simulink model "NUgus_servo"  (R2019a)
settings: Solver=VariableStepAuto  StartTime=0.0  StopTime=10  RelTol=1e-3
values from neighbouring files (symbols this model uses):
  head = [-0.05482228998067195, -0.00010888238321339966, 0.0011712900228573724, 0.41900000000000004]    [comtest.m]
  s = mean(abs(present_speed.data))    [RunServoTest.m]
  torso = [0.0050079703254699804, 0.008880921777563762, 0.1021503146237477, 2.5390000000000006]    [comtest.m]
undefined symbols (not defined in the file or in its folder): floor, X, Y, Z
libraries: sm_lib x206, fl_ps_legacy_lib x120, nesl_utility x62, fl_lib x8
(part 8 of 8)

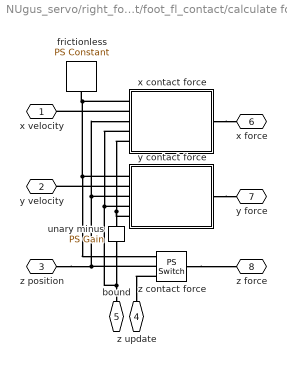
== system NUgus_servo/right_foot/foot_fl_contact/calculate forces ==
  frictionless : fl_lib/Physical Signals/Sources/PS Constant  constant=0
  unary minus : fl_ps_legacy_lib/Legacy Physical Signals/Functions/PS Gain  gain=-1
      settings: SourceProductName=Simscape
  x contact force : Subsystem
  y contact force : Subsystem
  z contact force : fl_ps_legacy_lib/Legacy Physical Signals/Nonlinear Operators/PS Switch  Threshold=0
      settings: SourceProductName=Simscape  SourceProductBaseCode=SS
  x velocity : PMIOPort  Side=Left
  y velocity : PMIOPort  Port=2  Side=Left
  z position : PMIOPort  Port=3  Side=Left
  z update : PMIOPort  Port=4  Side=Left
  bound : PMIOPort  Port=5  Side=Left
  x force : PMIOPort  Port=6  Side=Right
  y force : PMIOPort  Port=7  Side=Right
  z force : PMIOPort  Port=8  Side=Right
  connections:
  x contact force/LConn2 -- x velocity/RConn1
  y contact force/LConn2 -- y velocity/RConn1
  y contact force/RConn1 -- y force/RConn1
  x contact force/RConn1 -- x force/RConn1
  z contact force/RConn1 -- z force/RConn1
  y contact force/LConn3 -- x contact force/LConn3 -- z position/RConn1 -- z contact force/LConn2
  y contact force/LConn4 -- x contact force/LConn4 -- unary minus/LConn1 -- bound/RConn1
  y contact force/LConn5 -- x contact force/LConn5 -- unary minus/RConn1
  x contact force/LConn1 -- frictionless/RConn1 -- y contact force/LConn1 -- z contact force/LConn1
  z contact force/LConn3 -- z update/RConn1

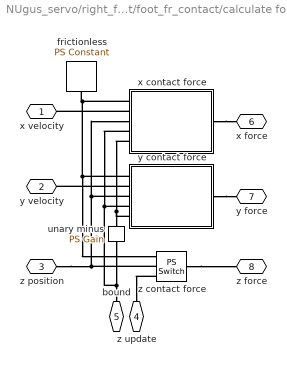
== system NUgus_servo/right_foot/foot_fr_contact/calculate forces ==
  frictionless : fl_lib/Physical Signals/Sources/PS Constant  constant=0
  unary minus : fl_ps_legacy_lib/Legacy Physical Signals/Functions/PS Gain  gain=-1
      settings: SourceProductName=Simscape
  x contact force : Subsystem
  y contact force : Subsystem
  z contact force : fl_ps_legacy_lib/Legacy Physical Signals/Nonlinear Operators/PS Switch  Threshold=0
      settings: SourceProductName=Simscape  SourceProductBaseCode=SS
  x velocity : PMIOPort  Side=Left
  y velocity : PMIOPort  Port=2  Side=Left
  z position : PMIOPort  Port=3  Side=Left
  z update : PMIOPort  Port=4  Side=Left
  bound : PMIOPort  Port=5  Side=Left
  x force : PMIOPort  Port=6  Side=Right
  y force : PMIOPort  Port=7  Side=Right
  z force : PMIOPort  Port=8  Side=Right
  connections:
  x contact force/LConn2 -- x velocity/RConn1
  y contact force/LConn2 -- y velocity/RConn1
  y contact force/RConn1 -- y force/RConn1
  x contact force/RConn1 -- x force/RConn1
  z contact force/RConn1 -- z force/RConn1
  y contact force/LConn3 -- x contact force/LConn3 -- z position/RConn1 -- z contact force/LConn2
  y contact force/LConn4 -- x contact force/LConn4 -- unary minus/LConn1 -- bound/RConn1
  y contact force/LConn5 -- x contact force/LConn5 -- unary minus/RConn1
  x contact force/LConn1 -- frictionless/RConn1 -- y contact force/LConn1 -- z contact force/LConn1
  z contact force/LConn3 -- z update/RConn1

== system NUgus_servo/left_foot/foot_bl_contact/calculate forces/x contact force ==
  PS Max : fl_ps_legacy_lib/Legacy Physical Signals/Nonlinear Operators/PS Max
      settings: SourceProductName=Simscape  SourceProductBaseCode=SS
  PS Min : fl_ps_legacy_lib/Legacy Physical Signals/Nonlinear Operators/PS Min
      settings: SourceProductName=Simscape  SourceProductBaseCode=SS
  PS Switch1 : fl_ps_legacy_lib/Legacy Physical Signals/Nonlinear Operators/PS Switch  Threshold=0
      settings: SourceProductName=Simscape  SourceProductBaseCode=SS
  frictionless : PMIOPort  Side=Left
  force : PMIOPort  Port=2  Side=Right
  velocity : PMIOPort  Port=3  Side=Left
  z position : PMIOPort  Port=4  Side=Left
  upper_bound : PMIOPort  Port=5  Side=Left
  lower_bound : PMIOPort  Port=6  Side=Left
  connections:
  PS Max/LConn2 -- lower_bound/RConn1
  PS Max/LConn1 -- PS Min/RConn1
  PS Switch1/LConn3 -- PS Max/RConn1
  PS Min/LConn1 -- velocity/RConn1
  z position/RConn1 -- PS Switch1/LConn2
  PS Switch1/LConn1 -- frictionless/RConn1
  PS Switch1/RConn1 -- force/RConn1
  PS Min/LConn2 -- upper_bound/RConn1

== system NUgus_servo/left_foot/foot_bl_contact/calculate forces/y contact force ==
  PS Max : fl_ps_legacy_lib/Legacy Physical Signals/Nonlinear Operators/PS Max
      settings: SourceProductName=Simscape  SourceProductBaseCode=SS
  PS Min : fl_ps_legacy_lib/Legacy Physical Signals/Nonlinear Operators/PS Min
      settings: SourceProductName=Simscape  SourceProductBaseCode=SS
  PS Switch1 : fl_ps_legacy_lib/Legacy Physical Signals/Nonlinear Operators/PS Switch  Threshold=0
      settings: SourceProductName=Simscape  SourceProductBaseCode=SS
  frictionless : PMIOPort  Side=Left
  force : PMIOPort  Port=2  Side=Right
  velocity : PMIOPort  Port=3  Side=Left
  z position : PMIOPort  Port=4  Side=Left
  upper_bound : PMIOPort  Port=5  Side=Left
  lower_bound : PMIOPort  Port=6  Side=Left
  connections:
  PS Max/LConn2 -- lower_bound/RConn1
  PS Max/LConn1 -- PS Min/RConn1
  PS Switch1/LConn3 -- PS Max/RConn1
  PS Min/LConn1 -- velocity/RConn1
  z position/RConn1 -- PS Switch1/LConn2
  PS Switch1/LConn1 -- frictionless/RConn1
  PS Switch1/RConn1 -- force/RConn1
  PS Min/LConn2 -- upper_bound/RConn1

== system NUgus_servo/left_foot/foot_br_contact/calculate forces/x contact force ==
  PS Max : fl_ps_legacy_lib/Legacy Physical Signals/Nonlinear Operators/PS Max
      settings: SourceProductName=Simscape  SourceProductBaseCode=SS
  PS Min : fl_ps_legacy_lib/Legacy Physical Signals/Nonlinear Operators/PS Min
      settings: SourceProductName=Simscape  SourceProductBaseCode=SS
  PS Switch1 : fl_ps_legacy_lib/Legacy Physical Signals/Nonlinear Operators/PS Switch  Threshold=0
      settings: SourceProductName=Simscape  SourceProductBaseCode=SS
  frictionless : PMIOPort  Side=Left
  force : PMIOPort  Port=2  Side=Right
  velocity : PMIOPort  Port=3  Side=Left
  z position : PMIOPort  Port=4  Side=Left
  upper_bound : PMIOPort  Port=5  Side=Left
  lower_bound : PMIOPort  Port=6  Side=Left
  connections:
  PS Max/LConn2 -- lower_bound/RConn1
  PS Max/LConn1 -- PS Min/RConn1
  PS Switch1/LConn3 -- PS Max/RConn1
  PS Min/LConn1 -- velocity/RConn1
  z position/RConn1 -- PS Switch1/LConn2
  PS Switch1/LConn1 -- frictionless/RConn1
  PS Switch1/RConn1 -- force/RConn1
  PS Min/LConn2 -- upper_bound/RConn1

== system NUgus_servo/left_foot/foot_br_contact/calculate forces/y contact force ==
  PS Max : fl_ps_legacy_lib/Legacy Physical Signals/Nonlinear Operators/PS Max
      settings: SourceProductName=Simscape  SourceProductBaseCode=SS
  PS Min : fl_ps_legacy_lib/Legacy Physical Signals/Nonlinear Operators/PS Min
      settings: SourceProductName=Simscape  SourceProductBaseCode=SS
  PS Switch1 : fl_ps_legacy_lib/Legacy Physical Signals/Nonlinear Operators/PS Switch  Threshold=0
      settings: SourceProductName=Simscape  SourceProductBaseCode=SS
  frictionless : PMIOPort  Side=Left
  force : PMIOPort  Port=2  Side=Right
  velocity : PMIOPort  Port=3  Side=Left
  z position : PMIOPort  Port=4  Side=Left
  upper_bound : PMIOPort  Port=5  Side=Left
  lower_bound : PMIOPort  Port=6  Side=Left
  connections:
  PS Max/LConn2 -- lower_bound/RConn1
  PS Max/LConn1 -- PS Min/RConn1
  PS Switch1/LConn3 -- PS Max/RConn1
  PS Min/LConn1 -- velocity/RConn1
  z position/RConn1 -- PS Switch1/LConn2
  PS Switch1/LConn1 -- frictionless/RConn1
  PS Switch1/RConn1 -- force/RConn1
  PS Min/LConn2 -- upper_bound/RConn1

== system NUgus_servo/left_foot/foot_fl_contact/calculate forces/x contact force ==
  PS Max : fl_ps_legacy_lib/Legacy Physical Signals/Nonlinear Operators/PS Max
      settings: SourceProductName=Simscape  SourceProductBaseCode=SS
  PS Min : fl_ps_legacy_lib/Legacy Physical Signals/Nonlinear Operators/PS Min
      settings: SourceProductName=Simscape  SourceProductBaseCode=SS
  PS Switch1 : fl_ps_legacy_lib/Legacy Physical Signals/Nonlinear Operators/PS Switch  Threshold=0
      settings: SourceProductName=Simscape  SourceProductBaseCode=SS
  frictionless : PMIOPort  Side=Left
  force : PMIOPort  Port=2  Side=Right
  velocity : PMIOPort  Port=3  Side=Left
  z position : PMIOPort  Port=4  Side=Left
  upper_bound : PMIOPort  Port=5  Side=Left
  lower_bound : PMIOPort  Port=6  Side=Left
  connections:
  PS Max/LConn2 -- lower_bound/RConn1
  PS Max/LConn1 -- PS Min/RConn1
  PS Switch1/LConn3 -- PS Max/RConn1
  PS Min/LConn1 -- velocity/RConn1
  z position/RConn1 -- PS Switch1/LConn2
  PS Switch1/LConn1 -- frictionless/RConn1
  PS Switch1/RConn1 -- force/RConn1
  PS Min/LConn2 -- upper_bound/RConn1

== system NUgus_servo/left_foot/foot_fl_contact/calculate forces/y contact force ==
  PS Max : fl_ps_legacy_lib/Legacy Physical Signals/Nonlinear Operators/PS Max
      settings: SourceProductName=Simscape  SourceProductBaseCode=SS
  PS Min : fl_ps_legacy_lib/Legacy Physical Signals/Nonlinear Operators/PS Min
      settings: SourceProductName=Simscape  SourceProductBaseCode=SS
  PS Switch1 : fl_ps_legacy_lib/Legacy Physical Signals/Nonlinear Operators/PS Switch  Threshold=0
      settings: SourceProductName=Simscape  SourceProductBaseCode=SS
  frictionless : PMIOPort  Side=Left
  force : PMIOPort  Port=2  Side=Right
  velocity : PMIOPort  Port=3  Side=Left
  z position : PMIOPort  Port=4  Side=Left
  upper_bound : PMIOPort  Port=5  Side=Left
  lower_bound : PMIOPort  Port=6  Side=Left
  connections:
  PS Max/LConn2 -- lower_bound/RConn1
  PS Max/LConn1 -- PS Min/RConn1
  PS Switch1/LConn3 -- PS Max/RConn1
  PS Min/LConn1 -- velocity/RConn1
  z position/RConn1 -- PS Switch1/LConn2
  PS Switch1/LConn1 -- frictionless/RConn1
  PS Switch1/RConn1 -- force/RConn1
  PS Min/LConn2 -- upper_bound/RConn1

== system NUgus_servo/left_foot/foot_fr_contact/calculate forces/x contact force ==
  PS Max : fl_ps_legacy_lib/Legacy Physical Signals/Nonlinear Operators/PS Max
      settings: SourceProductName=Simscape  SourceProductBaseCode=SS
  PS Min : fl_ps_legacy_lib/Legacy Physical Signals/Nonlinear Operators/PS Min
      settings: SourceProductName=Simscape  SourceProductBaseCode=SS
  PS Switch1 : fl_ps_legacy_lib/Legacy Physical Signals/Nonlinear Operators/PS Switch  Threshold=0
      settings: SourceProductName=Simscape  SourceProductBaseCode=SS
  frictionless : PMIOPort  Side=Left
  force : PMIOPort  Port=2  Side=Right
  velocity : PMIOPort  Port=3  Side=Left
  z position : PMIOPort  Port=4  Side=Left
  upper_bound : PMIOPort  Port=5  Side=Left
  lower_bound : PMIOPort  Port=6  Side=Left
  connections:
  PS Max/LConn2 -- lower_bound/RConn1
  PS Max/LConn1 -- PS Min/RConn1
  PS Switch1/LConn3 -- PS Max/RConn1
  PS Min/LConn1 -- velocity/RConn1
  z position/RConn1 -- PS Switch1/LConn2
  PS Switch1/LConn1 -- frictionless/RConn1
  PS Switch1/RConn1 -- force/RConn1
  PS Min/LConn2 -- upper_bound/RConn1

== system NUgus_servo/left_foot/foot_fr_contact/calculate forces/y contact force ==
  PS Max : fl_ps_legacy_lib/Legacy Physical Signals/Nonlinear Operators/PS Max
      settings: SourceProductName=Simscape  SourceProductBaseCode=SS
  PS Min : fl_ps_legacy_lib/Legacy Physical Signals/Nonlinear Operators/PS Min
      settings: SourceProductName=Simscape  SourceProductBaseCode=SS
  PS Switch1 : fl_ps_legacy_lib/Legacy Physical Signals/Nonlinear Operators/PS Switch  Threshold=0
      settings: SourceProductName=Simscape  SourceProductBaseCode=SS
  frictionless : PMIOPort  Side=Left
  force : PMIOPort  Port=2  Side=Right
  velocity : PMIOPort  Port=3  Side=Left
  z position : PMIOPort  Port=4  Side=Left
  upper_bound : PMIOPort  Port=5  Side=Left
  lower_bound : PMIOPort  Port=6  Side=Left
  connections:
  PS Max/LConn2 -- lower_bound/RConn1
  PS Max/LConn1 -- PS Min/RConn1
  PS Switch1/LConn3 -- PS Max/RConn1
  PS Min/LConn1 -- velocity/RConn1
  z position/RConn1 -- PS Switch1/LConn2
  PS Switch1/LConn1 -- frictionless/RConn1
  PS Switch1/RConn1 -- force/RConn1
  PS Min/LConn2 -- upper_bound/RConn1

== system NUgus_servo/right_foot/foot_bl_contact/calculate forces/x contact force ==
  PS Max : fl_ps_legacy_lib/Legacy Physical Signals/Nonlinear Operators/PS Max
      settings: SourceProductName=Simscape  SourceProductBaseCode=SS
  PS Min : fl_ps_legacy_lib/Legacy Physical Signals/Nonlinear Operators/PS Min
      settings: SourceProductName=Simscape  SourceProductBaseCode=SS
  PS Switch1 : fl_ps_legacy_lib/Legacy Physical Signals/Nonlinear Operators/PS Switch  Threshold=0
      settings: SourceProductName=Simscape  SourceProductBaseCode=SS
  frictionless : PMIOPort  Side=Left
  force : PMIOPort  Port=2  Side=Right
  velocity : PMIOPort  Port=3  Side=Left
  z position : PMIOPort  Port=4  Side=Left
  upper_bound : PMIOPort  Port=5  Side=Left
  lower_bound : PMIOPort  Port=6  Side=Left
  connections:
  PS Max/LConn2 -- lower_bound/RConn1
  PS Max/LConn1 -- PS Min/RConn1
  PS Switch1/LConn3 -- PS Max/RConn1
  PS Min/LConn1 -- velocity/RConn1
  z position/RConn1 -- PS Switch1/LConn2
  PS Switch1/LConn1 -- frictionless/RConn1
  PS Switch1/RConn1 -- force/RConn1
  PS Min/LConn2 -- upper_bound/RConn1

== system NUgus_servo/right_foot/foot_bl_contact/calculate forces/y contact force ==
  PS Max : fl_ps_legacy_lib/Legacy Physical Signals/Nonlinear Operators/PS Max
      settings: SourceProductName=Simscape  SourceProductBaseCode=SS
  PS Min : fl_ps_legacy_lib/Legacy Physical Signals/Nonlinear Operators/PS Min
      settings: SourceProductName=Simscape  SourceProductBaseCode=SS
  PS Switch1 : fl_ps_legacy_lib/Legacy Physical Signals/Nonlinear Operators/PS Switch  Threshold=0
      settings: SourceProductName=Simscape  SourceProductBaseCode=SS
  frictionless : PMIOPort  Side=Left
  force : PMIOPort  Port=2  Side=Right
  velocity : PMIOPort  Port=3  Side=Left
  z position : PMIOPort  Port=4  Side=Left
  upper_bound : PMIOPort  Port=5  Side=Left
  lower_bound : PMIOPort  Port=6  Side=Left
  connections:
  PS Max/LConn2 -- lower_bound/RConn1
  PS Max/LConn1 -- PS Min/RConn1
  PS Switch1/LConn3 -- PS Max/RConn1
  PS Min/LConn1 -- velocity/RConn1
  z position/RConn1 -- PS Switch1/LConn2
  PS Switch1/LConn1 -- frictionless/RConn1
  PS Switch1/RConn1 -- force/RConn1
  PS Min/LConn2 -- upper_bound/RConn1

== system NUgus_servo/right_foot/foot_br_contact/calculate forces/x contact force ==
  PS Max : fl_ps_legacy_lib/Legacy Physical Signals/Nonlinear Operators/PS Max
      settings: SourceProductName=Simscape  SourceProductBaseCode=SS
  PS Min : fl_ps_legacy_lib/Legacy Physical Signals/Nonlinear Operators/PS Min
      settings: SourceProductName=Simscape  SourceProductBaseCode=SS
  PS Switch1 : fl_ps_legacy_lib/Legacy Physical Signals/Nonlinear Operators/PS Switch  Threshold=0
      settings: SourceProductName=Simscape  SourceProductBaseCode=SS
  frictionless : PMIOPort  Side=Left
  force : PMIOPort  Port=2  Side=Right
  velocity : PMIOPort  Port=3  Side=Left
  z position : PMIOPort  Port=4  Side=Left
  upper_bound : PMIOPort  Port=5  Side=Left
  lower_bound : PMIOPort  Port=6  Side=Left
  connections:
  PS Max/LConn2 -- lower_bound/RConn1
  PS Max/LConn1 -- PS Min/RConn1
  PS Switch1/LConn3 -- PS Max/RConn1
  PS Min/LConn1 -- velocity/RConn1
  z position/RConn1 -- PS Switch1/LConn2
  PS Switch1/LConn1 -- frictionless/RConn1
  PS Switch1/RConn1 -- force/RConn1
  PS Min/LConn2 -- upper_bound/RConn1

== system NUgus_servo/right_foot/foot_br_contact/calculate forces/y contact force ==
  PS Max : fl_ps_legacy_lib/Legacy Physical Signals/Nonlinear Operators/PS Max
      settings: SourceProductName=Simscape  SourceProductBaseCode=SS
  PS Min : fl_ps_legacy_lib/Legacy Physical Signals/Nonlinear Operators/PS Min
      settings: SourceProductName=Simscape  SourceProductBaseCode=SS
  PS Switch1 : fl_ps_legacy_lib/Legacy Physical Signals/Nonlinear Operators/PS Switch  Threshold=0
      settings: SourceProductName=Simscape  SourceProductBaseCode=SS
  frictionless : PMIOPort  Side=Left
  force : PMIOPort  Port=2  Side=Right
  velocity : PMIOPort  Port=3  Side=Left
  z position : PMIOPort  Port=4  Side=Left
  upper_bound : PMIOPort  Port=5  Side=Left
  lower_bound : PMIOPort  Port=6  Side=Left
  connections:
  PS Max/LConn2 -- lower_bound/RConn1
  PS Max/LConn1 -- PS Min/RConn1
  PS Switch1/LConn3 -- PS Max/RConn1
  PS Min/LConn1 -- velocity/RConn1
  z position/RConn1 -- PS Switch1/LConn2
  PS Switch1/LConn1 -- frictionless/RConn1
  PS Switch1/RConn1 -- force/RConn1
  PS Min/LConn2 -- upper_bound/RConn1

== system NUgus_servo/right_foot/foot_fl_contact/calculate forces/x contact force ==
  PS Max : fl_ps_legacy_lib/Legacy Physical Signals/Nonlinear Operators/PS Max
      settings: SourceProductName=Simscape  SourceProductBaseCode=SS
  PS Min : fl_ps_legacy_lib/Legacy Physical Signals/Nonlinear Operators/PS Min
      settings: SourceProductName=Simscape  SourceProductBaseCode=SS
  PS Switch1 : fl_ps_legacy_lib/Legacy Physical Signals/Nonlinear Operators/PS Switch  Threshold=0
      settings: SourceProductName=Simscape  SourceProductBaseCode=SS
  frictionless : PMIOPort  Side=Left
  force : PMIOPort  Port=2  Side=Right
  velocity : PMIOPort  Port=3  Side=Left
  z position : PMIOPort  Port=4  Side=Left
  upper_bound : PMIOPort  Port=5  Side=Left
  lower_bound : PMIOPort  Port=6  Side=Left
  connections:
  PS Max/LConn2 -- lower_bound/RConn1
  PS Max/LConn1 -- PS Min/RConn1
  PS Switch1/LConn3 -- PS Max/RConn1
  PS Min/LConn1 -- velocity/RConn1
  z position/RConn1 -- PS Switch1/LConn2
  PS Switch1/LConn1 -- frictionless/RConn1
  PS Switch1/RConn1 -- force/RConn1
  PS Min/LConn2 -- upper_bound/RConn1

== system NUgus_servo/right_foot/foot_fl_contact/calculate forces/y contact force ==
  PS Max : fl_ps_legacy_lib/Legacy Physical Signals/Nonlinear Operators/PS Max
      settings: SourceProductName=Simscape  SourceProductBaseCode=SS
  PS Min : fl_ps_legacy_lib/Legacy Physical Signals/Nonlinear Operators/PS Min
      settings: SourceProductName=Simscape  SourceProductBaseCode=SS
  PS Switch1 : fl_ps_legacy_lib/Legacy Physical Signals/Nonlinear Operators/PS Switch  Threshold=0
      settings: SourceProductName=Simscape  SourceProductBaseCode=SS
  frictionless : PMIOPort  Side=Left
  force : PMIOPort  Port=2  Side=Right
  velocity : PMIOPort  Port=3  Side=Left
  z position : PMIOPort  Port=4  Side=Left
  upper_bound : PMIOPort  Port=5  Side=Left
  lower_bound : PMIOPort  Port=6  Side=Left
  connections:
  PS Max/LConn2 -- lower_bound/RConn1
  PS Max/LConn1 -- PS Min/RConn1
  PS Switch1/LConn3 -- PS Max/RConn1
  PS Min/LConn1 -- velocity/RConn1
  z position/RConn1 -- PS Switch1/LConn2
  PS Switch1/LConn1 -- frictionless/RConn1
  PS Switch1/RConn1 -- force/RConn1
  PS Min/LConn2 -- upper_bound/RConn1

== system NUgus_servo/right_foot/foot_fr_contact/calculate forces/x contact force ==
  PS Max : fl_ps_legacy_lib/Legacy Physical Signals/Nonlinear Operators/PS Max
      settings: SourceProductName=Simscape  SourceProductBaseCode=SS
  PS Min : fl_ps_legacy_lib/Legacy Physical Signals/Nonlinear Operators/PS Min
      settings: SourceProductName=Simscape  SourceProductBaseCode=SS
  PS Switch1 : fl_ps_legacy_lib/Legacy Physical Signals/Nonlinear Operators/PS Switch  Threshold=0
      settings: SourceProductName=Simscape  SourceProductBaseCode=SS
  frictionless : PMIOPort  Side=Left
  force : PMIOPort  Port=2  Side=Right
  velocity : PMIOPort  Port=3  Side=Left
  z position : PMIOPort  Port=4  Side=Left
  upper_bound : PMIOPort  Port=5  Side=Left
  lower_bound : PMIOPort  Port=6  Side=Left
  connections:
  PS Max/LConn2 -- lower_bound/RConn1
  PS Max/LConn1 -- PS Min/RConn1
  PS Switch1/LConn3 -- PS Max/RConn1
  PS Min/LConn1 -- velocity/RConn1
  z position/RConn1 -- PS Switch1/LConn2
  PS Switch1/LConn1 -- frictionless/RConn1
  PS Switch1/RConn1 -- force/RConn1
  PS Min/LConn2 -- upper_bound/RConn1

== system NUgus_servo/right_foot/foot_fr_contact/calculate forces/y contact force ==
  PS Max : fl_ps_legacy_lib/Legacy Physical Signals/Nonlinear Operators/PS Max
      settings: SourceProductName=Simscape  SourceProductBaseCode=SS
  PS Min : fl_ps_legacy_lib/Legacy Physical Signals/Nonlinear Operators/PS Min
      settings: SourceProductName=Simscape  SourceProductBaseCode=SS
  PS Switch1 : fl_ps_legacy_lib/Legacy Physical Signals/Nonlinear Operators/PS Switch  Threshold=0
      settings: SourceProductName=Simscape  SourceProductBaseCode=SS
  frictionless : PMIOPort  Side=Left
  force : PMIOPort  Port=2  Side=Right
  velocity : PMIOPort  Port=3  Side=Left
  z position : PMIOPort  Port=4  Side=Left
  upper_bound : PMIOPort  Port=5  Side=Left
  lower_bound : PMIOPort  Port=6  Side=Left
  connections:
  PS Max/LConn2 -- lower_bound/RConn1
  PS Max/LConn1 -- PS Min/RConn1
  PS Switch1/LConn3 -- PS Max/RConn1
  PS Min/LConn1 -- velocity/RConn1
  z position/RConn1 -- PS Switch1/LConn2
  PS Switch1/LConn1 -- frictionless/RConn1
  PS Switch1/RConn1 -- force/RConn1
  PS Min/LConn2 -- upper_bound/RConn1
